simulink model "PredictionPinson"  (R2019b)
settings: Solver=VariableStepAuto  StartTime=0.0  StopTime=36  RelTol=1e-3
settings Model: Creator=pieterpinson  LastModifiedBy=pieterpinson

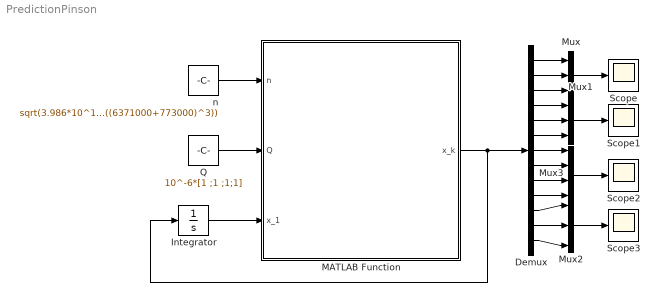
== system PredictionPinson ==
  Demux : Demux  Outputs=13
  Integrator : Integrator  InitialCondition=|  ContinuousStateAttributes='pose'
      | [-0.0019 ; 0.0017 ; 1.0891 ; 0 ; 0 ; 0 ; -0.7226 ; 0.6358 ; 0.1434 ; 0.2302
      | ; -0.0873 ; -0.1489 ; 0.0262]
  MATLAB Function : MATLAB Function  TreatAsAtomicUnit=on
  Mux : Mux  Inputs=3
  Mux1 : Mux  Inputs=3
  Mux2 : Mux  Inputs=3
  Mux3 : Mux
  Q : Constant  Value=10^-6*[1 ;1 ;1;1]
  Scope{,1..3} (4 alike) : Scope
  n : Constant  Value=sqrt(3.986*10^14/((6371000+773000)^3))
  wires:
  MATLAB Function/1(x_k) -> Integrator/1, Demux/1
  Integrator/1 -> MATLAB Function/3(x_1)
  Q/1 -> MATLAB Function/2(Q)
  n/1 -> MATLAB Function/1(n)
  Mux3/1 -> Scope2/1
  Demux/13 -> Mux2/3
  Demux/12 -> Mux2/2
  Demux/11 -> Mux2/1
  Demux/10 -> Mux3/4
  Demux/9 -> Mux3/3
  Demux/8 -> Mux3/2
  Demux/7 -> Mux3/1
  Demux/6 -> Mux1/3
  Demux/5 -> Mux1/2
  Demux/4 -> Mux1/1
  Demux/3 -> Mux/3
  Demux/2 -> Mux/2
  Demux/1 -> Mux/1
  Mux1/1 -> Scope1/1
  Mux/1 -> Scope/1
  Mux2/1 -> Scope3/1

== matlab function PredictionPinson/MATLAB Function ==
  data: n input; x_k output; Q input; x_1 input
function x_k = prediction(n,Q,x_1)

drr = [4-3*cos(n) 0 0 ; 6*(sin(n)-n) 1 0 ; 0 0 cos(n)];
drv = [sin(n)/n 2*(1-cos(n))/n 0 ; 2*(cos(n)-1)/n (4*sin(n)-3*n)/n 0 ; 0 0 sin(n)/n];
dvr = [3*n*sin(n) 0 0 ; 6*n*(cos(n)-1) 0 0 ; 0 0 -n*sin(n)];
dvv = [cos(n) 2*sin(n) 0 ; -2*sin(n) 4*cos(n)-3 0 ; 0 0 cos(n)]; 

dr = [drr drv];
dv = [dvr dvv];
fi_cw = [dr ; dv];

x_k = x_1;

x_k(1:6) = fi_cw*x_k(1:6);

x_k(7:10) = [0 x_1(13) -x_1(12) x_1(11) ; -x_1(13) 0 x_1(11) x_1(12) ; x_1(12) -x_1(11) 0 x_1(13) ; -x_1(11) -x_1(12) -x_1(13) 0]*normalize(x_1(7:10))/2 + Q;

end
